simulink model "Seat_Belt"  (R2025b)
settings: Solver=VariableStepAuto  StartTime=0.0  StopTime=inf  RelTol=1e-3
settings Model: Creator=Pai  LastModifiedBy=Pai

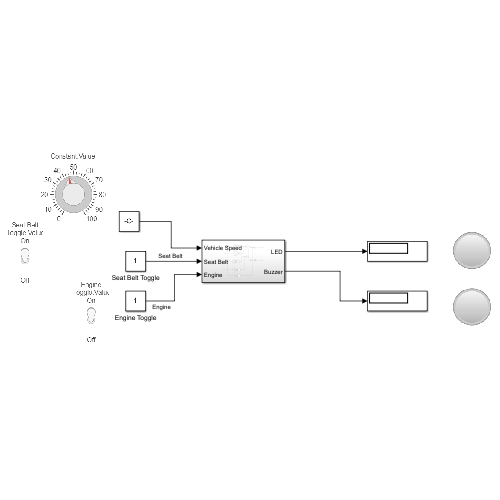
[thumbnail: Simulink's stored preview of the top-level diagram]
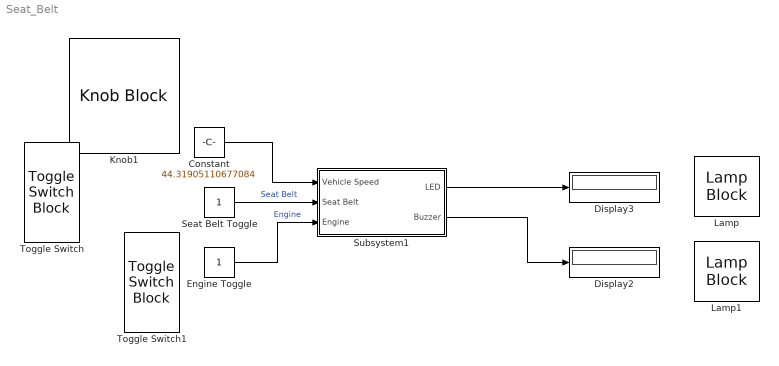
== system Seat_Belt ==
  Constant : Constant  Value=44.31905110677084
  Display2 : Display
  Display3 : Display
  Engine Toggle : Constant
  Knob1 : KnobBlock
  Lamp : LampBlock  LabelPosition=Hide  DefaultColor=[192.0, 192.0, 192.0]
  Lamp1 : LampBlock  LabelPosition=Hide  DefaultColor=[192.0, 192.0, 192.0]
  Seat Belt Toggle : Constant
  Subsystem1 : Subsystem
  Toggle Switch : ToggleSwitchBlock
  Toggle Switch1 : ToggleSwitchBlock
  wires:
  Seat Belt Toggle/1 -> Subsystem1/2(Seat Belt)  "Seat Belt"
  Engine Toggle/1 -> Subsystem1/3(Engine)  "Engine"
  Subsystem1/1(LED) -> Display3/1
  Subsystem1/2(Buzzer) -> Display2/1
  Constant/1 -> Subsystem1/1(Vehicle Speed)

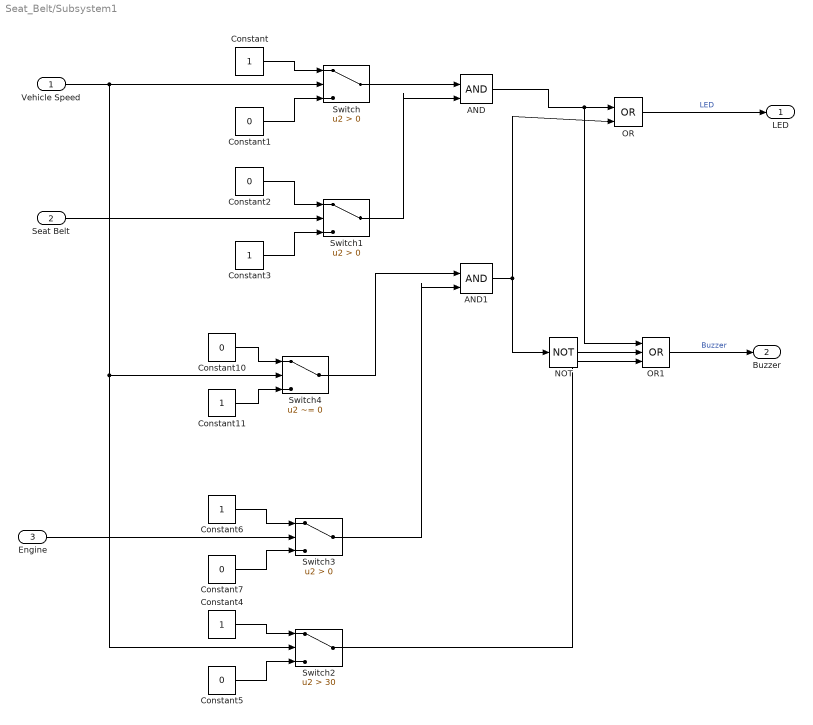
== system Seat_Belt/Subsystem1 ==
  Vehicle Speed : Inport
  Seat Belt : Inport  Port=2
  Engine : Inport  Port=3
  AND : Logic  IconShape=distinctive  AllPortsSameDT=off  OutDataTypeStr=boolean
  AND1 : Logic  IconShape=distinctive  AllPortsSameDT=off  OutDataTypeStr=boolean
  Constant{,3..4,6,11} (5 alike) : Constant
  Constant{1..2,5,7,10} (5 alike) : Constant  Value=0
  NOT : Logic  Operator=NOT  IconShape=distinctive  AllPortsSameDT=off  OutDataTypeStr=boolean
  OR : Logic  Operator=OR  IconShape=distinctive  AllPortsSameDT=off  OutDataTypeStr=boolean
  OR1 : Logic  Operator=OR  Inputs=3  IconShape=distinctive  AllPortsSameDT=off  OutDataTypeStr=boolean
  Switch : Switch  Criteria=u2 > Threshold  SaturateOnIntegerOverflow=off  InputSameDT=off
  Switch1 : Switch  Criteria=u2 > Threshold  SaturateOnIntegerOverflow=off  InputSameDT=off
  Switch2 : Switch  Criteria=u2 > Threshold  Threshold=30  SaturateOnIntegerOverflow=off  InputSameDT=off
  Switch3 : Switch  Criteria=u2 > Threshold  SaturateOnIntegerOverflow=off  InputSameDT=off
  Switch4 : Switch  Criteria=u2 ~= 0  SaturateOnIntegerOverflow=off  InputSameDT=off
  LED : Outport
  Buzzer : Outport  Port=2
  wires:
  Constant6/1 -> Switch3/1
  Vehicle Speed/1 -> Switch/2, Switch4/2, Switch2/2
  Constant3/1 -> Switch1/3
  Constant/1 -> Switch/1
  AND/1 -> OR1/1, OR/1
  OR1/1 -> Buzzer/1  "Buzzer"
  Switch/1 -> AND/1
  Constant2/1 -> Switch1/1
  Switch3/1 -> AND1/2
  Constant11/1 -> Switch4/3
  Constant10/1 -> Switch4/1
  Constant7/1 -> Switch3/3
  Constant4/1 -> Switch2/1
  Constant1/1 -> Switch/3
  Constant5/1 -> Switch2/3
  AND1/1 -> NOT/1, OR/2
  Switch2/1 -> OR1/3
  Switch4/1 -> AND1/1
  Seat Belt/1 -> Switch1/2
  OR/1 -> LED/1  "LED"
  Engine/1 -> Switch3/2
  Switch1/1 -> AND/2
  NOT/1 -> OR1/2
